simulink model "feedback_x"  (R2018b)
settings: Solver=VariableStepAuto  StartTime=0.0  StopTime=10  RelTol=1e-3
undefined symbols (not defined in the file): Ax, Ax_prime, Bx, Bx_prime, Cx, Cx_prime, Dx, Dx_prime, Kx, Sx, x0_chap, x0x
settings Model: Creator=Rafik  LastModifiedBy=Rafik

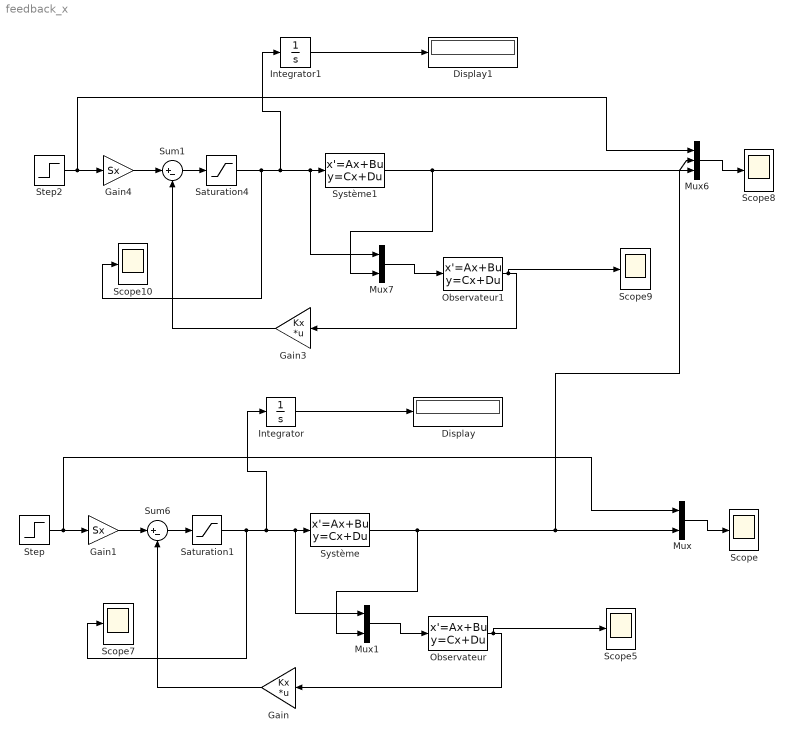
== system feedback_x ==
  Display : Display
  Display1 : Display
  Gain : Gain  Gain=Kx  Multiplication=Matrix(K*u)
  Gain1 : Gain  Gain=Sx
  Gain3 : Gain  Gain=Kx  Multiplication=Matrix(K*u)
  Gain4 : Gain  Gain=Sx
  Integrator : Integrator
  Integrator1 : Integrator
  Mux : Mux  Inputs=2
  Mux1 : Mux  Inputs=2
  Mux6 : Mux  Inputs=3
  Mux7 : Mux  Inputs=2
  Observateur : StateSpace  A=Ax_prime  B=Bx_prime  C=Cx_prime  D=Dx_prime  InitialCondition=x0_chap
  Observateur1 : StateSpace  A=Ax_prime  B=Bx_prime  C=Cx_prime  D=Dx_prime  InitialCondition=x0_chap
  Saturation1 : Saturate  UpperLimit=110  LowerLimit=-110
  Saturation4 : Saturate  UpperLimit=110  LowerLimit=-110
  Scope{,5,7..10} (6 alike) : Scope
  Step : Step  Time=0  After=0.5  SampleTime=0
  Step2 : Step  Time=0  After=0.5  SampleTime=0
  Sum1 : Sum  Inputs=|+-
  Sum6 : Sum  Inputs=|+-
  Système : StateSpace  A=Ax  B=Bx  C=Cx  D=Dx  InitialCondition=x0x
  Système1 : StateSpace  A=|  B=Bx  C=Cx  D=Dx  InitialCondition=x0x
      | [-0.8635   -0.3450
      | ;    1.2500         0]
  wires:
  Mux/1 -> Scope/1
  Système/1 -> Mux6/3, Mux/2, Mux1/2
  Mux1/1 -> Observateur/1
  Gain/1 -> Sum6/2
  Step/1 -> Mux/1, Gain1/1
  Observateur/1 -> Scope5/1, Gain/1
  Gain1/1 -> Sum6/1
  Sum6/1 -> Saturation1/1
  Saturation1/1 -> Scope7/1, Integrator/1, Mux1/1, Système/1
  Integrator/1 -> Display/1
  Integrator1/1 -> Display1/1
  Gain4/1 -> Sum1/1
  Saturation4/1 -> Scope10/1, Integrator1/1, Mux7/1, Système1/1
  Sum1/1 -> Saturation4/1
  Observateur1/1 -> Scope9/1, Gain3/1
  Gain3/1 -> Sum1/2
  Step2/1 -> Mux6/1, Gain4/1
  Système1/1 -> Mux6/2, Mux7/2
  Mux7/1 -> Observateur1/1
  Mux6/1 -> Scope8/1
